simulink model "SecRwRtStHdrstUpwdDnwdTrgtPosSelc"  (R2018b)
settings: Solver=FixedStepDiscrete  StartTime=0.0  StopTime=10.0  FixedStep=0.01  RelTol=1e-3
undefined symbols (not defined in the file or in its folder): KeSMSw4SAcsMd23SecRwRtStHdrstUpwdDnwdPos_Val, KeSMSw4SAcsMd23SecRwRtStHdrstUpwdDnwdPosMax_Val, KeSMSw4SAcsMd23SecRwRtStHdrstUpwdDnwdPosMin_Val, KeSMSw4SAcsMd24SecRwRtStHdrstUpwdDnwdPos_Val, KeSMSw4SAcsMd24SecRwRtStHdrstUpwdDnwdPosMax_Val, KeSMSw4SAcsMd24SecRwRtStHdrstUpwdDnwdPosMin_Val, KeSMSw4SAcsMd25SecRwRtStHdrstUpwdDnwdPos_Val, KeSMSw4SAcsMd25SecRwRtStHdrstUpwdDnwdPosMax_Val, KeSMSw4SAcsMd25SecRwRtStHdrstUpwdDnwdPosMin_Val, KeSMSw4SAcsMd26SecRwRtStHdrstUpwdDnwdPos_Val, KeSMSw4SAcsMd26SecRwRtStHdrstUpwdDnwdPosMax_Val, KeSMSw4SAcsMd26SecRwRtStHdrstUpwdDnwdPosMin_Val, KeSMSw4sLyingMDSecRwRtStHdrstUpwdPos_160_Val, KeSMSw4sLyingMDSecRwRtStHdrstUpwdPos_165_Val, KeSMSw4sLyingMDSecRwRtStHdrstUpwdPos_170_Val, KeSMSw4sLyingMDSecRwRtStHdrstUpwdPos_175_Val, KeSMSw4sLyingMDSecRwRtStHdrstUpwdPos_180_Val, KeSMSw4sLyingMDSecRwRtStHdrstUpwdPos_Below160_Val, KeSMSw4sLyingMDSecRwRtStHdrstUpwdPos_Over180_Val, KeSMSw4sLyingMDSecRwRtStHdrstUpwdPosMax_160_Val, KeSMSw4sLyingMDSecRwRtStHdrstUpwdPosMax_165_Val, KeSMSw4sLyingMDSecRwRtStHdrstUpwdPosMax_170_Val, KeSMSw4sLyingMDSecRwRtStHdrstUpwdPosMax_175_Val, KeSMSw4sLyingMDSecRwRtStHdrstUpwdPosMax_180_Val, KeSMSw4sLyingMDSecRwRtStHdrstUpwdPosMax_Below160_Val, KeSMSw4sLyingMDSecRwRtStHdrstUpwdPosMax_Over180_Val, KeSMSw4sLyingMDSecRwRtStHdrstUpwdPosMin_160_Val, KeSMSw4sLyingMDSecRwRtStHdrstUpwdPosMin_165_Val, KeSMSw4sLyingMDSecRwRtStHdrstUpwdPosMin_170_Val, KeSMSw4sLyingMDSecRwRtStHdrstUpwdPosMin_175_Val, KeSMSw4sLyingMDSecRwRtStHdrstUpwdPosMin_180_Val, KeSMSw4sLyingMDSecRwRtStHdrstUpwdPosMin_Below160_Val, KeSMSw4sLyingMDSecRwRtStHdrstUpwdPosMin_Over180_Val, KeSMSw4sRecoveryMDSecRwRtStHdrstUpwdPos_160_Val, KeSMSw4sRecoveryMDSecRwRtStHdrstUpwdPos_165_Val, KeSMSw4sRecoveryMDSecRwRtStHdrstUpwdPos_170_Val, KeSMSw4sRecoveryMDSecRwRtStHdrstUpwdPos_175_Val, KeSMSw4sRecoveryMDSecRwRtStHdrstUpwdPos_180_Val, KeSMSw4sRecoveryMDSecRwRtStHdrstUpwdPos_Below160_Val, KeSMSw4sRecoveryMDSecRwRtStHdrstUpwdPos_Over180_Val, KeSMSw4sRecoveryMDSecRwRtStHdrstUpwdPosMax_160_Val, KeSMSw4sRecoveryMDSecRwRtStHdrstUpwdPosMax_165_Val, KeSMSw4sRecoveryMDSecRwRtStHdrstUpwdPosMax_170_Val, KeSMSw4sRecoveryMDSecRwRtStHdrstUpwdPosMax_175_Val, KeSMSw4sRecoveryMDSecRwRtStHdrstUpwdPosMax_180_Val, KeSMSw4sRecoveryMDSecRwRtStHdrstUpwdPosMax_Below160_Val, KeSMSw4sRecoveryMDSecRwRtStHdrstUpwdPosMax_Over180_Val, KeSMSw4sRecoveryMDSecRwRtStHdrstUpwdPosMin_160_Val, KeSMSw4sRecoveryMDSecRwRtStHdrstUpwdPosMin_165_Val, KeSMSw4sRecoveryMDSecRwRtStHdrstUpwdPosMin_170_Val, KeSMSw4sRecoveryMDSecRwRtStHdrstUpwdPosMin_175_Val, KeSMSw4sRecoveryMDSecRwRtStHdrstUpwdPosMin_180_Val, KeSMSw4sRecoveryMDSecRwRtStHdrstUpwdPosMin_Below160_Val, KeSMSw4sRecoveryMDSecRwRtStHdrstUpwdPosMin_Over180_Val, KeSMSw4sVIPMDSecRwRtStHdrstUpwdPos_160_Val, KeSMSw4sVIPMDSecRwRtStHdrstUpwdPos_165_Val, KeSMSw4sVIPMDSecRwRtStHdrstUpwdPos_170_Val, KeSMSw4sVIPMDSecRwRtStHdrstUpwdPos_175_Val, KeSMSw4sVIPMDSecRwRtStHdrstUpwdPos_180_Val, KeSMSw4sVIPMDSecRwRtStHdrstUpwdPos_Below160_Val ... (+15)
libraries: TrgtPosSelcLib x4
settings Model: ModifiedHistory=2023.8.1 V2.0.0 CR421790 增加模式21-26  Creator=sn2xws  LastModifiedBy=sn2xws
settings DataIOCC: SaveFormat=StructureWithTime
settings OptimizationCC: DefaultParameterBehavior=Inlined  EnhancedBackFolding=on  PassReuseOutputArgsAs=Individual arguments  ZeroExternalMemoryAtStartup=off  ZeroInternalMemoryAtStartup=off  OptimizeBlockOrder=speed  DifferentSizesBufferReuse=on  OptimizationCustomize=off
settings DebuggingCC: ParameterTunabilityLossMsg=error
settings ModelReferenceCC: ModelReferenceNumInstancesAllowed=Single
settings SFSimCC: MATLABDynamicMemAlloc=off
settings RTWCC: SystemTargetFile=autosar.tlc  GenCodeOnly=on  TemplateMakefile=ert_default_tmf  Description=AUTOSAR  GenerateReport=on  IncludeHyperlinkInReport=on  LaunchReport=on  GenerateTraceInfo=on  GenerateTraceReport=on  GenerateTraceReportSl=on  GenerateTraceReportSf=on  GenerateTraceReportEml=on
settings CodeAppCC: ForceParamTrailComments=on  IgnoreCustomStorageClasses=off  OperatorAnnotations=on  SimulinkDataObjDesc=on  SFDataObjDesc=on  InsertBlockDesc=on
settings STFCustomTargetCC: TargetLangStandard=C99 (ISO)  MultiwordLength=256  ParMdlRefBuildCompliant=on  CompOptLevelCompliant=on  IncludeMdlTerminateFcn=off  CombineOutputUpdateFcns=on  SuppressErrorStatus=on  ERTCustomFileBanners=on  SupportNonFinite=off  SupportComplex=off  SupportContinuousTime=off  SupportNonInlinedSFcns=off  RemoveResetFunc=on  MATLABClassNameForMDSCustomization=Simulink.SoftwareTarget.ERTCustomization  AutosarCompliant=on  UseToolchainInfoCompliant=on  LookupTableObjectStructAxisOrder=2,1,3,4,...  LUTObjectStructOrderEvenSpacing=Size,Table,Breakpoints  SystemTargetFile=autosar.tlc
settings ERTTargetCC: TargetLangStandard=C99 (ISO)  ConcurrentExecutionCompliant=off  IncludeMdlTerminateFcn=off  SuppressErrorStatus=on  SupportNonFinite=off  SupportComplex=off  ModelStepFunctionPrototypeControlCompliant=off  CPPClassGenCompliant=off  AutosarCompliant=on  LookupTableObjectStructAxisOrder=2,1,3,4,...  LUTObjectStructOrderEvenSpacing=Size,Table,Breakpoints  InlinedParameterPlacement=NonHierarchical  ERTCustomFileTemplate=example_file_process.tlc  ERTFilePackagingFormat=Compact

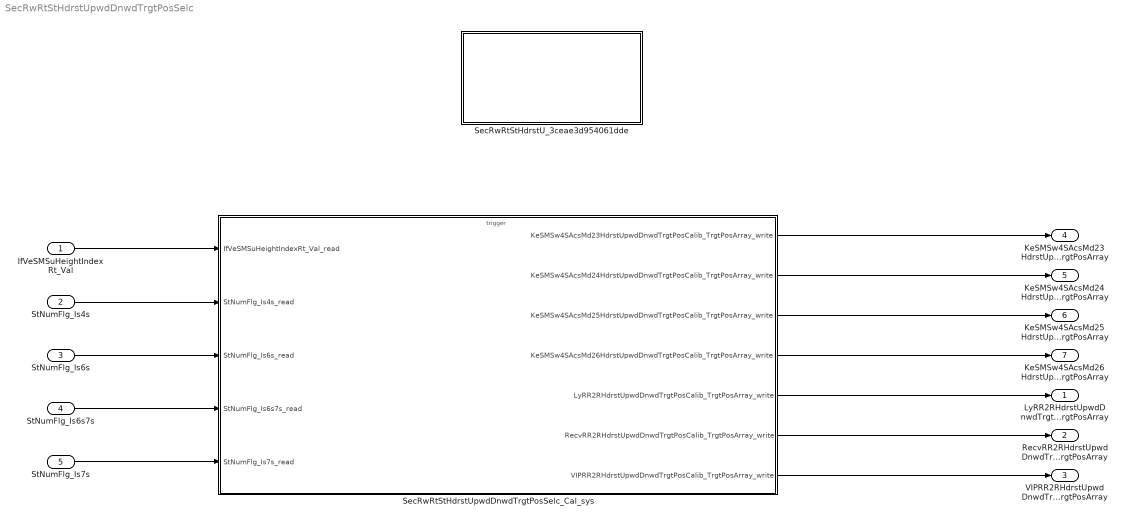
== system SecRwRtStHdrstUpwdDnwdTrgtPosSelc ==
  IfVeSMSuHeightIndexRt_Val : Inport  Description=|  OutDataTypeStr=uint8  PortDimensions=1
      | 0：under 160
      | 1：160
      | 2：165
      | 3：170
      | 4：175
      | 5：180
      | 6：over 180
  StNumFlg_Is4s : Inport  Port=2  OutDataTypeStr=boolean  PortDimensions=1
  StNumFlg_Is6s : Inport  Port=3  OutDataTypeStr=boolean  PortDimensions=1
  StNumFlg_Is6s7s : Inport  Port=4  OutDataTypeStr=boolean  PortDimensions=1
  StNumFlg_Is7s : Inport  Port=5  OutDataTypeStr=boolean  PortDimensions=1
  SecRwRtStHdrstU_3ceae3d954061dde : Subsystem
  SecRwRtStHdrstUpwdDnwdTrgtPosSelc_Cal_sys : Subsystem
  LyRR2RHdrstUpwdDnwdTrgtPosCalib_TrgtPosArray : Outport  Description=|  OutDataTypeStr=uint16  PortDimensions=3
      | 0:Pos
      | 1:Max
      | 2:Min
  RecvRR2RHdrstUpwdDnwdTrgtPosCalib_TrgtPosArray : Outport  Description=|  Port=2  OutDataTypeStr=uint16  PortDimensions=3
      | 0:Pos
      | 1:Max
      | 2:Min
  VIPRR2RHdrstUpwdDnwdTrgtPosCalib_TrgtPosArray : Outport  Description=|  Port=3  OutDataTypeStr=uint16  PortDimensions=3
      | 0:Pos
      | 1:Max
      | 2:Min
  KeSMSw4SAcsMd23HdrstUpwdDnwdTrgtPosCalib_TrgtPosArray : Outport  Description=|  Port=4  OutDataTypeStr=uint16  PortDimensions=3
      | 0:Pos
      | 1:Max
      | 2:Min
  KeSMSw4SAcsMd24HdrstUpwdDnwdTrgtPosCalib_TrgtPosArray : Outport  Description=|  Port=5  OutDataTypeStr=uint16  PortDimensions=3
      | 0:Pos
      | 1:Max
      | 2:Min
  KeSMSw4SAcsMd25HdrstUpwdDnwdTrgtPosCalib_TrgtPosArray : Outport  Description=|  Port=6  OutDataTypeStr=uint16  PortDimensions=3
      | 0:Pos
      | 1:Max
      | 2:Min
  KeSMSw4SAcsMd26HdrstUpwdDnwdTrgtPosCalib_TrgtPosArray : Outport  Description=|  Port=7  OutDataTypeStr=uint16  PortDimensions=3
      | 0:Pos
      | 1:Max
      | 2:Min
  wires:
  IfVeSMSuHeightIndexRt_Val/1 -> SecRwRtStHdrstUpwdDnwdTrgtPosSelc_Cal_sys/1(IfVeSMSuHeightIndexRt_Val_read)
  StNumFlg_Is4s/1 -> SecRwRtStHdrstUpwdDnwdTrgtPosSelc_Cal_sys/2(StNumFlg_Is4s_read)
  StNumFlg_Is6s/1 -> SecRwRtStHdrstUpwdDnwdTrgtPosSelc_Cal_sys/3(StNumFlg_Is6s_read)
  StNumFlg_Is6s7s/1 -> SecRwRtStHdrstUpwdDnwdTrgtPosSelc_Cal_sys/4(StNumFlg_Is6s7s_read)
  StNumFlg_Is7s/1 -> SecRwRtStHdrstUpwdDnwdTrgtPosSelc_Cal_sys/5(StNumFlg_Is7s_read)
  SecRwRtStHdrstUpwdDnwdTrgtPosSelc_Cal_sys/5(LyRR2RHdrstUpwdDnwdTrgtPosCalib_TrgtPosArray_write) -> LyRR2RHdrstUpwdDnwdTrgtPosCalib_TrgtPosArray/1
  SecRwRtStHdrstUpwdDnwdTrgtPosSelc_Cal_sys/6(RecvRR2RHdrstUpwdDnwdTrgtPosCalib_TrgtPosArray_write) -> RecvRR2RHdrstUpwdDnwdTrgtPosCalib_TrgtPosArray/1
  SecRwRtStHdrstUpwdDnwdTrgtPosSelc_Cal_sys/7(VIPRR2RHdrstUpwdDnwdTrgtPosCalib_TrgtPosArray_write) -> VIPRR2RHdrstUpwdDnwdTrgtPosCalib_TrgtPosArray/1
  SecRwRtStHdrstUpwdDnwdTrgtPosSelc_Cal_sys/1(KeSMSw4SAcsMd23HdrstUpwdDnwdTrgtPosCalib_TrgtPosArray_write) -> KeSMSw4SAcsMd23HdrstUpwdDnwdTrgtPosCalib_TrgtPosArray/1
  SecRwRtStHdrstUpwdDnwdTrgtPosSelc_Cal_sys/2(KeSMSw4SAcsMd24HdrstUpwdDnwdTrgtPosCalib_TrgtPosArray_write) -> KeSMSw4SAcsMd24HdrstUpwdDnwdTrgtPosCalib_TrgtPosArray/1
  SecRwRtStHdrstUpwdDnwdTrgtPosSelc_Cal_sys/3(KeSMSw4SAcsMd25HdrstUpwdDnwdTrgtPosCalib_TrgtPosArray_write) -> KeSMSw4SAcsMd25HdrstUpwdDnwdTrgtPosCalib_TrgtPosArray/1
  SecRwRtStHdrstUpwdDnwdTrgtPosSelc_Cal_sys/4(KeSMSw4SAcsMd26HdrstUpwdDnwdTrgtPosCalib_TrgtPosArray_write) -> KeSMSw4SAcsMd26HdrstUpwdDnwdTrgtPosCalib_TrgtPosArray/1

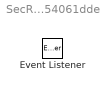
== system SecRwRtStHdrstUpwdDnwdTrgtPosSelc/SecRwRtStHdrstU_3ceae3d954061dde ==
  Event Listener : EventListener  EventName=reset

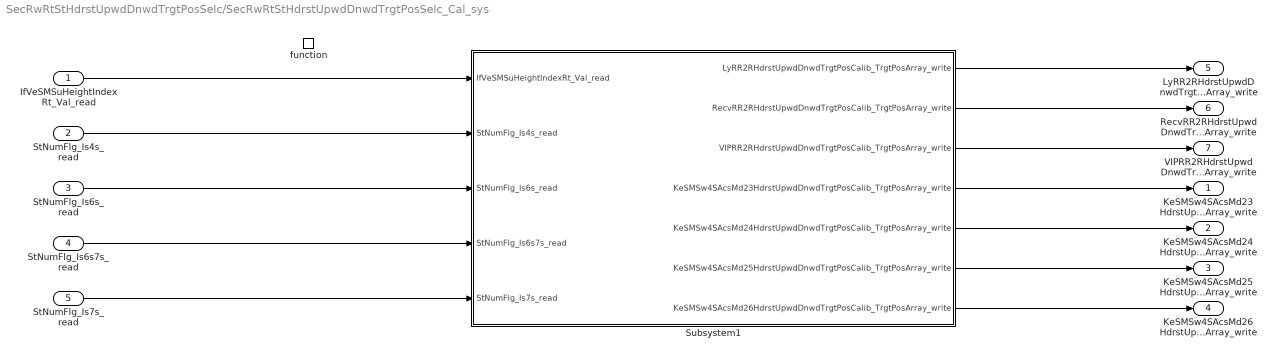
== system SecRwRtStHdrstUpwdDnwdTrgtPosSelc/SecRwRtStHdrstUpwdDnwdTrgtPosSelc_Cal_sys ==
  IfVeSMSuHeightIndexRt_Val_read : Inport
  StNumFlg_Is4s_read : Inport  Port=2
  StNumFlg_Is6s_read : Inport  Port=3
  StNumFlg_Is6s7s_read : Inport  Port=4
  StNumFlg_Is7s_read : Inport  Port=5
  function : TriggerPort  TriggerType=function-call  IsSimulinkFunction=on  FunctionName=SecRwRtStHdrstUpwdDnwdTrgtPosSelc_Cal  VariantControl=(inherit)
  Subsystem1 : Subsystem
  KeSMSw4SAcsMd23HdrstUpwdDnwdTrgtPosCalib_TrgtPosArray_write : Outport
      settings: EnsureOutportIsVirtual=on
  KeSMSw4SAcsMd24HdrstUpwdDnwdTrgtPosCalib_TrgtPosArray_write : Outport  Port=2
      settings: EnsureOutportIsVirtual=on
  KeSMSw4SAcsMd25HdrstUpwdDnwdTrgtPosCalib_TrgtPosArray_write : Outport  Port=3
      settings: EnsureOutportIsVirtual=on
  KeSMSw4SAcsMd26HdrstUpwdDnwdTrgtPosCalib_TrgtPosArray_write : Outport  Port=4
      settings: EnsureOutportIsVirtual=on
  LyRR2RHdrstUpwdDnwdTrgtPosCalib_TrgtPosArray_write : Outport  Port=5
      settings: EnsureOutportIsVirtual=on
  RecvRR2RHdrstUpwdDnwdTrgtPosCalib_TrgtPosArray_write : Outport  Port=6
      settings: EnsureOutportIsVirtual=on
  VIPRR2RHdrstUpwdDnwdTrgtPosCalib_TrgtPosArray_write : Outport  Port=7
      settings: EnsureOutportIsVirtual=on
  wires:
  Subsystem1/1(LyRR2RHdrstUpwdDnwdTrgtPosCalib_TrgtPosArray_write) -> LyRR2RHdrstUpwdDnwdTrgtPosCalib_TrgtPosArray_write/1
  Subsystem1/2(RecvRR2RHdrstUpwdDnwdTrgtPosCalib_TrgtPosArray_write) -> RecvRR2RHdrstUpwdDnwdTrgtPosCalib_TrgtPosArray_write/1
  Subsystem1/3(VIPRR2RHdrstUpwdDnwdTrgtPosCalib_TrgtPosArray_write) -> VIPRR2RHdrstUpwdDnwdTrgtPosCalib_TrgtPosArray_write/1
  Subsystem1/4(KeSMSw4SAcsMd23HdrstUpwdDnwdTrgtPosCalib_TrgtPosArray_write) -> KeSMSw4SAcsMd23HdrstUpwdDnwdTrgtPosCalib_TrgtPosArray_write/1
  Subsystem1/5(KeSMSw4SAcsMd24HdrstUpwdDnwdTrgtPosCalib_TrgtPosArray_write) -> KeSMSw4SAcsMd24HdrstUpwdDnwdTrgtPosCalib_TrgtPosArray_write/1
  Subsystem1/6(KeSMSw4SAcsMd25HdrstUpwdDnwdTrgtPosCalib_TrgtPosArray_write) -> KeSMSw4SAcsMd25HdrstUpwdDnwdTrgtPosCalib_TrgtPosArray_write/1
  Subsystem1/7(KeSMSw4SAcsMd26HdrstUpwdDnwdTrgtPosCalib_TrgtPosArray_write) -> KeSMSw4SAcsMd26HdrstUpwdDnwdTrgtPosCalib_TrgtPosArray_write/1
  StNumFlg_Is6s7s_read/1 -> Subsystem1/4(StNumFlg_Is6s7s_read)
  StNumFlg_Is6s_read/1 -> Subsystem1/3(StNumFlg_Is6s_read)
  StNumFlg_Is7s_read/1 -> Subsystem1/5(StNumFlg_Is7s_read)
  StNumFlg_Is4s_read/1 -> Subsystem1/2(StNumFlg_Is4s_read)
  IfVeSMSuHeightIndexRt_Val_read/1 -> Subsystem1/1(IfVeSMSuHeightIndexRt_Val_read)

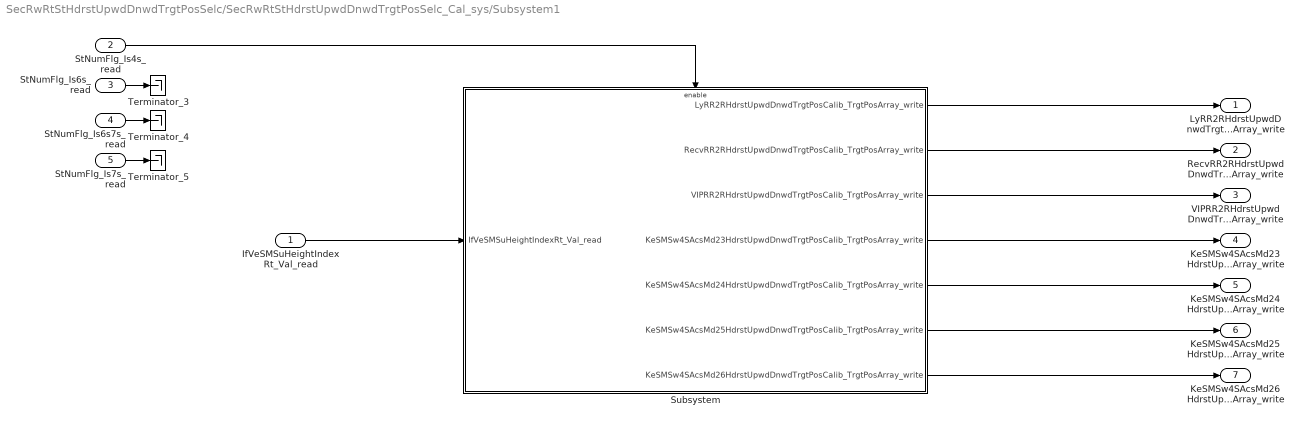
== system SecRwRtStHdrstUpwdDnwdTrgtPosSelc/SecRwRtStHdrstUpwdDnwdTrgtPosSelc_Cal_sys/Subsystem1 ==
  IfVeSMSuHeightIndexRt_Val_read : Inport
  StNumFlg_Is4s_read : Inport  Port=2
  StNumFlg_Is6s_read : Inport  Port=3
  StNumFlg_Is6s7s_read : Inport  Port=4
  StNumFlg_Is7s_read : Inport  Port=5
  Subsystem : Subsystem
  Terminator_3 : Terminator
  Terminator_4 : Terminator
  Terminator_5 : Terminator
  LyRR2RHdrstUpwdDnwdTrgtPosCalib_TrgtPosArray_write : Outport
      settings: EnsureOutportIsVirtual=on
  RecvRR2RHdrstUpwdDnwdTrgtPosCalib_TrgtPosArray_write : Outport  Port=2
      settings: EnsureOutportIsVirtual=on
  VIPRR2RHdrstUpwdDnwdTrgtPosCalib_TrgtPosArray_write : Outport  Port=3
      settings: EnsureOutportIsVirtual=on
  KeSMSw4SAcsMd23HdrstUpwdDnwdTrgtPosCalib_TrgtPosArray_write : Outport  Port=4
      settings: EnsureOutportIsVirtual=on
  KeSMSw4SAcsMd24HdrstUpwdDnwdTrgtPosCalib_TrgtPosArray_write : Outport  Port=5
      settings: EnsureOutportIsVirtual=on
  KeSMSw4SAcsMd25HdrstUpwdDnwdTrgtPosCalib_TrgtPosArray_write : Outport  Port=6
      settings: EnsureOutportIsVirtual=on
  KeSMSw4SAcsMd26HdrstUpwdDnwdTrgtPosCalib_TrgtPosArray_write : Outport  Port=7
      settings: EnsureOutportIsVirtual=on
  wires:
  Subsystem/3(VIPRR2RHdrstUpwdDnwdTrgtPosCalib_TrgtPosArray_write) -> VIPRR2RHdrstUpwdDnwdTrgtPosCalib_TrgtPosArray_write/1
  IfVeSMSuHeightIndexRt_Val_read/1 -> Subsystem/1(IfVeSMSuHeightIndexRt_Val_read)
  StNumFlg_Is4s_read/1 -> Subsystem/Enable
  StNumFlg_Is7s_read/1 -> Terminator_5/1
  StNumFlg_Is6s_read/1 -> Terminator_3/1
  StNumFlg_Is6s7s_read/1 -> Terminator_4/1
  Subsystem/2(RecvRR2RHdrstUpwdDnwdTrgtPosCalib_TrgtPosArray_write) -> RecvRR2RHdrstUpwdDnwdTrgtPosCalib_TrgtPosArray_write/1
  Subsystem/1(LyRR2RHdrstUpwdDnwdTrgtPosCalib_TrgtPosArray_write) -> LyRR2RHdrstUpwdDnwdTrgtPosCalib_TrgtPosArray_write/1
  Subsystem/4(KeSMSw4SAcsMd23HdrstUpwdDnwdTrgtPosCalib_TrgtPosArray_write) -> KeSMSw4SAcsMd23HdrstUpwdDnwdTrgtPosCalib_TrgtPosArray_write/1
  Subsystem/5(KeSMSw4SAcsMd24HdrstUpwdDnwdTrgtPosCalib_TrgtPosArray_write) -> KeSMSw4SAcsMd24HdrstUpwdDnwdTrgtPosCalib_TrgtPosArray_write/1
  Subsystem/6(KeSMSw4SAcsMd25HdrstUpwdDnwdTrgtPosCalib_TrgtPosArray_write) -> KeSMSw4SAcsMd25HdrstUpwdDnwdTrgtPosCalib_TrgtPosArray_write/1
  Subsystem/7(KeSMSw4SAcsMd26HdrstUpwdDnwdTrgtPosCalib_TrgtPosArray_write) -> KeSMSw4SAcsMd26HdrstUpwdDnwdTrgtPosCalib_TrgtPosArray_write/1

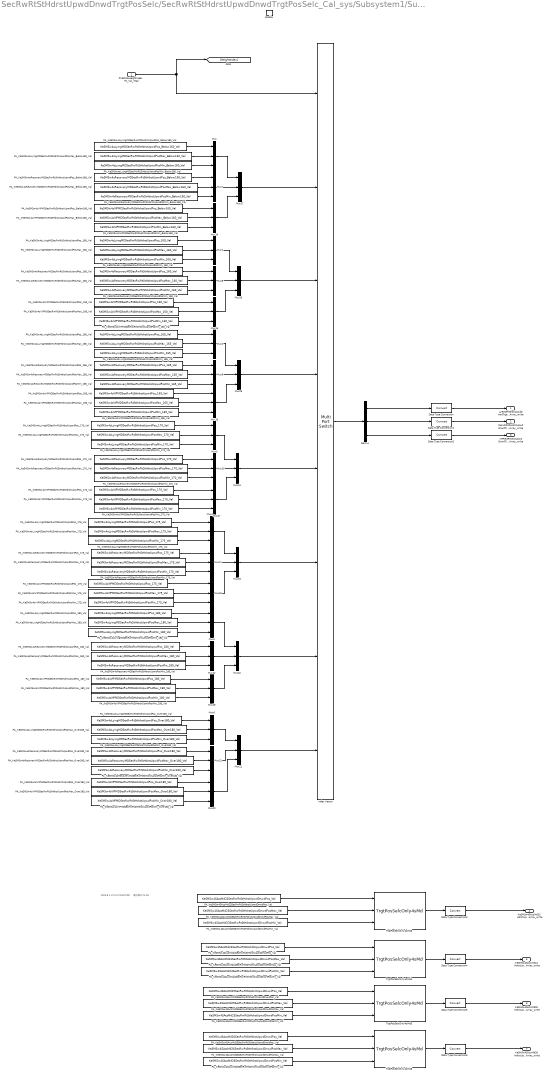
== system SecRwRtStHdrstUpwdDnwdTrgtPosSelc/SecRwRtStHdrstUpwdDnwdTrgtPosSelc_Cal_sys/Subsystem1/Subsystem ==
  note: 2023.8.1 V2.0.0 CR401790 增加模式21-26
  IfVeSMSuHeightIndexRt_Val_read : Inport
  Enable : EnablePort
  Data Type Conversion{,1..6} (7 alike) : DataTypeConversion
  Demux : Demux  Outputs=3
  Index Vector : MultiPortSwitch  DataPortOrder=Zero-based contiguous  Inputs=7  zeroidx=on
  Mux{,1..27} (28 alike) : Mux  Inputs=3
  PA_KeSMSw4SAcsMd23SecRwRtStHdrstUpwdDnwdPosMax_Val : Constant  Value=KeSMSw4SAcsMd23SecRwRtStHdrstUpwdDnwdPosMax_Val
  PA_KeSMSw4SAcsMd23SecRwRtStHdrstUpwdDnwdPosMin_Val : Constant  Value=KeSMSw4SAcsMd23SecRwRtStHdrstUpwdDnwdPosMin_Val
  PA_KeSMSw4SAcsMd23SecRwRtStHdrstUpwdDnwdPos_Val : Constant  Value=KeSMSw4SAcsMd23SecRwRtStHdrstUpwdDnwdPos_Val
  PA_KeSMSw4SAcsMd24SecRwRtStHdrstUpwdDnwdPosMax_Val : Constant  Value=KeSMSw4SAcsMd24SecRwRtStHdrstUpwdDnwdPosMax_Val
  PA_KeSMSw4SAcsMd24SecRwRtStHdrstUpwdDnwdPosMin_Val : Constant  Value=KeSMSw4SAcsMd24SecRwRtStHdrstUpwdDnwdPosMin_Val
  PA_KeSMSw4SAcsMd24SecRwRtStHdrstUpwdDnwdPos_Val : Constant  Value=KeSMSw4SAcsMd24SecRwRtStHdrstUpwdDnwdPos_Val
  PA_KeSMSw4SAcsMd25SecRwRtStHdrstUpwdDnwdPosMax_Val : Constant  Value=KeSMSw4SAcsMd25SecRwRtStHdrstUpwdDnwdPosMax_Val
  PA_KeSMSw4SAcsMd25SecRwRtStHdrstUpwdDnwdPosMin_Val : Constant  Value=KeSMSw4SAcsMd25SecRwRtStHdrstUpwdDnwdPosMin_Val
  PA_KeSMSw4SAcsMd25SecRwRtStHdrstUpwdDnwdPos_Val : Constant  Value=KeSMSw4SAcsMd25SecRwRtStHdrstUpwdDnwdPos_Val
  PA_KeSMSw4SAcsMd26SecRwRtStHdrstUpwdDnwdPosMax_Val : Constant  Value=KeSMSw4SAcsMd26SecRwRtStHdrstUpwdDnwdPosMax_Val
  PA_KeSMSw4SAcsMd26SecRwRtStHdrstUpwdDnwdPosMin_Val : Constant  Value=KeSMSw4SAcsMd26SecRwRtStHdrstUpwdDnwdPosMin_Val
  PA_KeSMSw4SAcsMd26SecRwRtStHdrstUpwdDnwdPos_Val : Constant  Value=KeSMSw4SAcsMd26SecRwRtStHdrstUpwdDnwdPos_Val
  PA_KeSMSw4sLyingMDSecRwRtStHdrstUpwdPosMax_160_Val : Constant  Value=KeSMSw4sLyingMDSecRwRtStHdrstUpwdPosMax_160_Val
  PA_KeSMSw4sLyingMDSecRwRtStHdrstUpwdPosMax_165_Val : Constant  Value=KeSMSw4sLyingMDSecRwRtStHdrstUpwdPosMax_165_Val
  PA_KeSMSw4sLyingMDSecRwRtStHdrstUpwdPosMax_170_Val : Constant  Value=KeSMSw4sLyingMDSecRwRtStHdrstUpwdPosMax_170_Val
  PA_KeSMSw4sLyingMDSecRwRtStHdrstUpwdPosMax_175_Val : Constant  Value=KeSMSw4sLyingMDSecRwRtStHdrstUpwdPosMax_175_Val
  PA_KeSMSw4sLyingMDSecRwRtStHdrstUpwdPosMax_180_Val : Constant  Value=KeSMSw4sLyingMDSecRwRtStHdrstUpwdPosMax_180_Val
  PA_KeSMSw4sLyingMDSecRwRtStHdrstUpwdPosMax_Below160_Val : Constant  Value=KeSMSw4sLyingMDSecRwRtStHdrstUpwdPosMax_Below160_Val
  PA_KeSMSw4sLyingMDSecRwRtStHdrstUpwdPosMax_Over180_Val : Constant  Value=KeSMSw4sLyingMDSecRwRtStHdrstUpwdPosMax_Over180_Val
  PA_KeSMSw4sLyingMDSecRwRtStHdrstUpwdPosMin_160_Val : Constant  Value=KeSMSw4sLyingMDSecRwRtStHdrstUpwdPosMin_160_Val
  PA_KeSMSw4sLyingMDSecRwRtStHdrstUpwdPosMin_165_Val : Constant  Value=KeSMSw4sLyingMDSecRwRtStHdrstUpwdPosMin_165_Val
  PA_KeSMSw4sLyingMDSecRwRtStHdrstUpwdPosMin_170_Val : Constant  Value=KeSMSw4sLyingMDSecRwRtStHdrstUpwdPosMin_170_Val
  PA_KeSMSw4sLyingMDSecRwRtStHdrstUpwdPosMin_175_Val : Constant  Value=KeSMSw4sLyingMDSecRwRtStHdrstUpwdPosMin_175_Val
  PA_KeSMSw4sLyingMDSecRwRtStHdrstUpwdPosMin_180_Val : Constant  Value=KeSMSw4sLyingMDSecRwRtStHdrstUpwdPosMin_180_Val
  PA_KeSMSw4sLyingMDSecRwRtStHdrstUpwdPosMin_Below160_Val : Constant  Value=KeSMSw4sLyingMDSecRwRtStHdrstUpwdPosMin_Below160_Val
  PA_KeSMSw4sLyingMDSecRwRtStHdrstUpwdPosMin_Over180_Val : Constant  Value=KeSMSw4sLyingMDSecRwRtStHdrstUpwdPosMin_Over180_Val
  PA_KeSMSw4sLyingMDSecRwRtStHdrstUpwdPos_160_Val : Constant  Value=KeSMSw4sLyingMDSecRwRtStHdrstUpwdPos_160_Val
  PA_KeSMSw4sLyingMDSecRwRtStHdrstUpwdPos_165_Val : Constant  Value=KeSMSw4sLyingMDSecRwRtStHdrstUpwdPos_165_Val
  PA_KeSMSw4sLyingMDSecRwRtStHdrstUpwdPos_170_Val : Constant  Value=KeSMSw4sLyingMDSecRwRtStHdrstUpwdPos_170_Val
  PA_KeSMSw4sLyingMDSecRwRtStHdrstUpwdPos_175_Val : Constant  Value=KeSMSw4sLyingMDSecRwRtStHdrstUpwdPos_175_Val
  PA_KeSMSw4sLyingMDSecRwRtStHdrstUpwdPos_180_Val : Constant  Value=KeSMSw4sLyingMDSecRwRtStHdrstUpwdPos_180_Val
  PA_KeSMSw4sLyingMDSecRwRtStHdrstUpwdPos_Below160_Val : Constant  Value=KeSMSw4sLyingMDSecRwRtStHdrstUpwdPos_Below160_Val
  PA_KeSMSw4sLyingMDSecRwRtStHdrstUpwdPos_Over180_Val : Constant  Value=KeSMSw4sLyingMDSecRwRtStHdrstUpwdPos_Over180_Val
  PA_KeSMSw4sRecoveryMDSecRwRtStHdrstUpwdPosMax_160_Val : Constant  Value=KeSMSw4sRecoveryMDSecRwRtStHdrstUpwdPosMax_160_Val
  PA_KeSMSw4sRecoveryMDSecRwRtStHdrstUpwdPosMax_165_Val : Constant  Value=KeSMSw4sRecoveryMDSecRwRtStHdrstUpwdPosMax_165_Val
  PA_KeSMSw4sRecoveryMDSecRwRtStHdrstUpwdPosMax_170_Val : Constant  Value=KeSMSw4sRecoveryMDSecRwRtStHdrstUpwdPosMax_170_Val
  PA_KeSMSw4sRecoveryMDSecRwRtStHdrstUpwdPosMax_175_Val : Constant  Value=KeSMSw4sRecoveryMDSecRwRtStHdrstUpwdPosMax_175_Val
  PA_KeSMSw4sRecoveryMDSecRwRtStHdrstUpwdPosMax_180_Val : Constant  Value=KeSMSw4sRecoveryMDSecRwRtStHdrstUpwdPosMax_180_Val
  PA_KeSMSw4sRecoveryMDSecRwRtStHdrstUpwdPosMax_Below160_Val : Constant  Value=KeSMSw4sRecoveryMDSecRwRtStHdrstUpwdPosMax_Below160_Val
  PA_KeSMSw4sRecoveryMDSecRwRtStHdrstUpwdPosMax_Over180_Val : Constant  Value=KeSMSw4sRecoveryMDSecRwRtStHdrstUpwdPosMax_Over180_Val
  PA_KeSMSw4sRecoveryMDSecRwRtStHdrstUpwdPosMin_160_Val : Constant  Value=KeSMSw4sRecoveryMDSecRwRtStHdrstUpwdPosMin_160_Val
  PA_KeSMSw4sRecoveryMDSecRwRtStHdrstUpwdPosMin_165_Val : Constant  Value=KeSMSw4sRecoveryMDSecRwRtStHdrstUpwdPosMin_165_Val
  PA_KeSMSw4sRecoveryMDSecRwRtStHdrstUpwdPosMin_170_Val : Constant  Value=KeSMSw4sRecoveryMDSecRwRtStHdrstUpwdPosMin_170_Val
  PA_KeSMSw4sRecoveryMDSecRwRtStHdrstUpwdPosMin_175_Val : Constant  Value=KeSMSw4sRecoveryMDSecRwRtStHdrstUpwdPosMin_175_Val
  PA_KeSMSw4sRecoveryMDSecRwRtStHdrstUpwdPosMin_180_Val : Constant  Value=KeSMSw4sRecoveryMDSecRwRtStHdrstUpwdPosMin_180_Val
  PA_KeSMSw4sRecoveryMDSecRwRtStHdrstUpwdPosMin_Below160_Val : Constant  Value=KeSMSw4sRecoveryMDSecRwRtStHdrstUpwdPosMin_Below160_Val
  PA_KeSMSw4sRecoveryMDSecRwRtStHdrstUpwdPosMin_Over180_Val : Constant  Value=KeSMSw4sRecoveryMDSecRwRtStHdrstUpwdPosMin_Over180_Val
  PA_KeSMSw4sRecoveryMDSecRwRtStHdrstUpwdPos_160_Val : Constant  Value=KeSMSw4sRecoveryMDSecRwRtStHdrstUpwdPos_160_Val
  PA_KeSMSw4sRecoveryMDSecRwRtStHdrstUpwdPos_165_Val : Constant  Value=KeSMSw4sRecoveryMDSecRwRtStHdrstUpwdPos_165_Val
  PA_KeSMSw4sRecoveryMDSecRwRtStHdrstUpwdPos_170_Val : Constant  Value=KeSMSw4sRecoveryMDSecRwRtStHdrstUpwdPos_170_Val
  PA_KeSMSw4sRecoveryMDSecRwRtStHdrstUpwdPos_175_Val : Constant  Value=KeSMSw4sRecoveryMDSecRwRtStHdrstUpwdPos_175_Val
  PA_KeSMSw4sRecoveryMDSecRwRtStHdrstUpwdPos_180_Val : Constant  Value=KeSMSw4sRecoveryMDSecRwRtStHdrstUpwdPos_180_Val
  PA_KeSMSw4sRecoveryMDSecRwRtStHdrstUpwdPos_Below160_Val : Constant  Value=KeSMSw4sRecoveryMDSecRwRtStHdrstUpwdPos_Below160_Val
  PA_KeSMSw4sRecoveryMDSecRwRtStHdrstUpwdPos_Over180_Val : Constant  Value=KeSMSw4sRecoveryMDSecRwRtStHdrstUpwdPos_Over180_Val
  PA_KeSMSw4sVIPMDSecRwRtStHdrstUpwdPosMax_160_Val : Constant  Value=KeSMSw4sVIPMDSecRwRtStHdrstUpwdPosMax_160_Val
  PA_KeSMSw4sVIPMDSecRwRtStHdrstUpwdPosMax_165_Val : Constant  Value=KeSMSw4sVIPMDSecRwRtStHdrstUpwdPosMax_165_Val
  PA_KeSMSw4sVIPMDSecRwRtStHdrstUpwdPosMax_170_Val : Constant  Value=KeSMSw4sVIPMDSecRwRtStHdrstUpwdPosMax_170_Val
  PA_KeSMSw4sVIPMDSecRwRtStHdrstUpwdPosMax_175_Val : Constant  Value=KeSMSw4sVIPMDSecRwRtStHdrstUpwdPosMax_175_Val
  PA_KeSMSw4sVIPMDSecRwRtStHdrstUpwdPosMax_180_Val : Constant  Value=KeSMSw4sVIPMDSecRwRtStHdrstUpwdPosMax_180_Val
  PA_KeSMSw4sVIPMDSecRwRtStHdrstUpwdPosMax_Below160_Val : Constant  Value=KeSMSw4sVIPMDSecRwRtStHdrstUpwdPosMax_Below160_Val
  PA_KeSMSw4sVIPMDSecRwRtStHdrstUpwdPosMax_Over180_Val : Constant  Value=KeSMSw4sVIPMDSecRwRtStHdrstUpwdPosMax_Over180_Val
  PA_KeSMSw4sVIPMDSecRwRtStHdrstUpwdPosMin_160_Val : Constant  Value=KeSMSw4sVIPMDSecRwRtStHdrstUpwdPosMin_160_Val
  PA_KeSMSw4sVIPMDSecRwRtStHdrstUpwdPosMin_165_Val : Constant  Value=KeSMSw4sVIPMDSecRwRtStHdrstUpwdPosMin_165_Val
  PA_KeSMSw4sVIPMDSecRwRtStHdrstUpwdPosMin_170_Val : Constant  Value=KeSMSw4sVIPMDSecRwRtStHdrstUpwdPosMin_170_Val
  PA_KeSMSw4sVIPMDSecRwRtStHdrstUpwdPosMin_175_Val : Constant  Value=KeSMSw4sVIPMDSecRwRtStHdrstUpwdPosMin_175_Val
  PA_KeSMSw4sVIPMDSecRwRtStHdrstUpwdPosMin_180_Val : Constant  Value=KeSMSw4sVIPMDSecRwRtStHdrstUpwdPosMin_180_Val
  PA_KeSMSw4sVIPMDSecRwRtStHdrstUpwdPosMin_Below160_Val : Constant  Value=KeSMSw4sVIPMDSecRwRtStHdrstUpwdPosMin_Below160_Val
  PA_KeSMSw4sVIPMDSecRwRtStHdrstUpwdPosMin_Over180_Val : Constant  Value=KeSMSw4sVIPMDSecRwRtStHdrstUpwdPosMin_Over180_Val
  PA_KeSMSw4sVIPMDSecRwRtStHdrstUpwdPos_160_Val : Constant  Value=KeSMSw4sVIPMDSecRwRtStHdrstUpwdPos_160_Val
  PA_KeSMSw4sVIPMDSecRwRtStHdrstUpwdPos_165_Val : Constant  Value=KeSMSw4sVIPMDSecRwRtStHdrstUpwdPos_165_Val
  PA_KeSMSw4sVIPMDSecRwRtStHdrstUpwdPos_170_Val : Constant  Value=KeSMSw4sVIPMDSecRwRtStHdrstUpwdPos_170_Val
  PA_KeSMSw4sVIPMDSecRwRtStHdrstUpwdPos_175_Val : Constant  Value=KeSMSw4sVIPMDSecRwRtStHdrstUpwdPos_175_Val
  PA_KeSMSw4sVIPMDSecRwRtStHdrstUpwdPos_180_Val : Constant  Value=KeSMSw4sVIPMDSecRwRtStHdrstUpwdPos_180_Val
  PA_KeSMSw4sVIPMDSecRwRtStHdrstUpwdPos_Below160_Val : Constant  Value=KeSMSw4sVIPMDSecRwRtStHdrstUpwdPos_Below160_Val
  PA_KeSMSw4sVIPMDSecRwRtStHdrstUpwdPos_Over180_Val : Constant  Value=KeSMSw4sVIPMDSecRwRtStHdrstUpwdPos_Over180_Val
  TrgtPosSelcOnly4sMd{3..6} (4 alike) : TrgtPosSelcLib/TrgtPosSelcOnly4sMd  SystemSampleTime=-1
  LyRR2RHdrstUpwdDnwdTrgtPosCalib_TrgtPosArray_write : Outport
  RecvRR2RHdrstUpwdDnwdTrgtPosCalib_TrgtPosArray_write : Outport  Port=2
  VIPRR2RHdrstUpwdDnwdTrgtPosCalib_TrgtPosArray_write : Outport  Port=3
  KeSMSw4SAcsMd23HdrstUpwdDnwdTrgtPosCalib_TrgtPosArray_write : Outport  Port=4
  KeSMSw4SAcsMd24HdrstUpwdDnwdTrgtPosCalib_TrgtPosArray_write : Outport  Port=5
  KeSMSw4SAcsMd25HdrstUpwdDnwdTrgtPosCalib_TrgtPosArray_write : Outport  Port=6
  KeSMSw4SAcsMd26HdrstUpwdDnwdTrgtPosCalib_TrgtPosArray_write : Outport  Port=7
  wires:
  Demux/1 -> Data Type Conversion/1
  IfVeSMSuHeightIndexRt_Val_read/1 -> [HeightIndex], Index Vector/1
  Demux/2 -> Data Type Conversion1/1
  Demux/3 -> Data Type Conversion2/1
  Data Type Conversion/1 -> LyRR2RHdrstUpwdDnwdTrgtPosCalib_TrgtPosArray_write/1
  Data Type Conversion1/1 -> RecvRR2RHdrstUpwdDnwdTrgtPosCalib_TrgtPosArray_write/1
  Data Type Conversion2/1 -> VIPRR2RHdrstUpwdDnwdTrgtPosCalib_TrgtPosArray_write/1
  PA_KeSMSw4SAcsMd23SecRwRtStHdrstUpwdDnwdPos_Val/1 -> TrgtPosSelcOnly4sMd3/1
  PA_KeSMSw4SAcsMd24SecRwRtStHdrstUpwdDnwdPos_Val/1 -> TrgtPosSelcOnly4sMd4/1
  PA_KeSMSw4SAcsMd25SecRwRtStHdrstUpwdDnwdPos_Val/1 -> TrgtPosSelcOnly4sMd5/1
  PA_KeSMSw4SAcsMd26SecRwRtStHdrstUpwdDnwdPos_Val/1 -> TrgtPosSelcOnly4sMd6/1
  TrgtPosSelcOnly4sMd5/1 -> Data Type Conversion5/1
  TrgtPosSelcOnly4sMd6/1 -> Data Type Conversion6/1
  TrgtPosSelcOnly4sMd3/1 -> Data Type Conversion3/1
  TrgtPosSelcOnly4sMd4/1 -> Data Type Conversion4/1
  PA_KeSMSw4SAcsMd23SecRwRtStHdrstUpwdDnwdPosMax_Val/1 -> TrgtPosSelcOnly4sMd3/2
  PA_KeSMSw4SAcsMd23SecRwRtStHdrstUpwdDnwdPosMin_Val/1 -> TrgtPosSelcOnly4sMd3/3
  PA_KeSMSw4SAcsMd24SecRwRtStHdrstUpwdDnwdPosMax_Val/1 -> TrgtPosSelcOnly4sMd4/2
  PA_KeSMSw4SAcsMd24SecRwRtStHdrstUpwdDnwdPosMin_Val/1 -> TrgtPosSelcOnly4sMd4/3
  PA_KeSMSw4SAcsMd25SecRwRtStHdrstUpwdDnwdPosMax_Val/1 -> TrgtPosSelcOnly4sMd5/2
  PA_KeSMSw4SAcsMd25SecRwRtStHdrstUpwdDnwdPosMin_Val/1 -> TrgtPosSelcOnly4sMd5/3
  PA_KeSMSw4SAcsMd26SecRwRtStHdrstUpwdDnwdPosMax_Val/1 -> TrgtPosSelcOnly4sMd6/2
  PA_KeSMSw4SAcsMd26SecRwRtStHdrstUpwdDnwdPosMin_Val/1 -> TrgtPosSelcOnly4sMd6/3
  Data Type Conversion3/1 -> KeSMSw4SAcsMd23HdrstUpwdDnwdTrgtPosCalib_TrgtPosArray_write/1
  Data Type Conversion4/1 -> KeSMSw4SAcsMd24HdrstUpwdDnwdTrgtPosCalib_TrgtPosArray_write/1
  Data Type Conversion5/1 -> KeSMSw4SAcsMd25HdrstUpwdDnwdTrgtPosCalib_TrgtPosArray_write/1
  Data Type Conversion6/1 -> KeSMSw4SAcsMd26HdrstUpwdDnwdTrgtPosCalib_TrgtPosArray_write/1
  PA_KeSMSw4sLyingMDSecRwRtStHdrstUpwdPos_Below160_Val/1 -> Mux/1
  PA_KeSMSw4sLyingMDSecRwRtStHdrstUpwdPosMax_Below160_Val/1 -> Mux/2
  PA_KeSMSw4sLyingMDSecRwRtStHdrstUpwdPosMin_Below160_Val/1 -> Mux/3
  PA_KeSMSw4sLyingMDSecRwRtStHdrstUpwdPosMax_160_Val/1 -> Mux1/2
  PA_KeSMSw4sLyingMDSecRwRtStHdrstUpwdPosMin_160_Val/1 -> Mux1/3
  PA_KeSMSw4sLyingMDSecRwRtStHdrstUpwdPos_160_Val/1 -> Mux1/1
  PA_KeSMSw4sLyingMDSecRwRtStHdrstUpwdPosMax_165_Val/1 -> Mux2/2
  PA_KeSMSw4sLyingMDSecRwRtStHdrstUpwdPosMin_165_Val/1 -> Mux2/3
  PA_KeSMSw4sLyingMDSecRwRtStHdrstUpwdPos_165_Val/1 -> Mux2/1
  PA_KeSMSw4sLyingMDSecRwRtStHdrstUpwdPosMax_170_Val/1 -> Mux3/2
  PA_KeSMSw4sLyingMDSecRwRtStHdrstUpwdPosMin_170_Val/1 -> Mux3/3
  PA_KeSMSw4sLyingMDSecRwRtStHdrstUpwdPos_170_Val/1 -> Mux3/1
  PA_KeSMSw4sLyingMDSecRwRtStHdrstUpwdPosMax_175_Val/1 -> Mux4/2
  PA_KeSMSw4sLyingMDSecRwRtStHdrstUpwdPosMin_175_Val/1 -> Mux4/3
  PA_KeSMSw4sLyingMDSecRwRtStHdrstUpwdPos_175_Val/1 -> Mux4/1
  PA_KeSMSw4sLyingMDSecRwRtStHdrstUpwdPosMax_180_Val/1 -> Mux5/2
  PA_KeSMSw4sLyingMDSecRwRtStHdrstUpwdPos_180_Val/1 -> Mux5/1
  PA_KeSMSw4sLyingMDSecRwRtStHdrstUpwdPosMin_180_Val/1 -> Mux5/3
  PA_KeSMSw4sLyingMDSecRwRtStHdrstUpwdPosMax_Over180_Val/1 -> Mux6/2
  PA_KeSMSw4sLyingMDSecRwRtStHdrstUpwdPosMin_Over180_Val/1 -> Mux6/3
  PA_KeSMSw4sLyingMDSecRwRtStHdrstUpwdPos_Over180_Val/1 -> Mux6/1
  PA_KeSMSw4sRecoveryMDSecRwRtStHdrstUpwdPosMax_Below160_Val/1 -> Mux7/2
  PA_KeSMSw4sRecoveryMDSecRwRtStHdrstUpwdPosMin_Below160_Val/1 -> Mux7/3
  PA_KeSMSw4sRecoveryMDSecRwRtStHdrstUpwdPos_Below160_Val/1 -> Mux7/1
  PA_KeSMSw4sRecoveryMDSecRwRtStHdrstUpwdPosMax_160_Val/1 -> Mux8/2
  PA_KeSMSw4sRecoveryMDSecRwRtStHdrstUpwdPosMin_160_Val/1 -> Mux8/3
  PA_KeSMSw4sRecoveryMDSecRwRtStHdrstUpwdPos_160_Val/1 -> Mux8/1
  PA_KeSMSw4sRecoveryMDSecRwRtStHdrstUpwdPosMax_165_Val/1 -> Mux9/2
  PA_KeSMSw4sRecoveryMDSecRwRtStHdrstUpwdPosMin_165_Val/1 -> Mux9/3
  PA_KeSMSw4sRecoveryMDSecRwRtStHdrstUpwdPos_165_Val/1 -> Mux9/1
  PA_KeSMSw4sRecoveryMDSecRwRtStHdrstUpwdPosMax_170_Val/1 -> Mux10/2
  PA_KeSMSw4sRecoveryMDSecRwRtStHdrstUpwdPosMin_170_Val/1 -> Mux10/3
  PA_KeSMSw4sRecoveryMDSecRwRtStHdrstUpwdPos_170_Val/1 -> Mux10/1
  PA_KeSMSw4sRecoveryMDSecRwRtStHdrstUpwdPosMax_175_Val/1 -> Mux11/2
  PA_KeSMSw4sRecoveryMDSecRwRtStHdrstUpwdPosMin_175_Val/1 -> Mux11/3
  PA_KeSMSw4sRecoveryMDSecRwRtStHdrstUpwdPos_175_Val/1 -> Mux11/1
  PA_KeSMSw4sRecoveryMDSecRwRtStHdrstUpwdPosMax_180_Val/1 -> Mux12/2
  PA_KeSMSw4sRecoveryMDSecRwRtStHdrstUpwdPosMin_180_Val/1 -> Mux12/3
  PA_KeSMSw4sRecoveryMDSecRwRtStHdrstUpwdPos_180_Val/1 -> Mux12/1
  PA_KeSMSw4sRecoveryMDSecRwRtStHdrstUpwdPosMax_Over180_Val/1 -> Mux13/2
  PA_KeSMSw4sRecoveryMDSecRwRtStHdrstUpwdPosMin_Over180_Val/1 -> Mux13/3
  PA_KeSMSw4sRecoveryMDSecRwRtStHdrstUpwdPos_Over180_Val/1 -> Mux13/1
  PA_KeSMSw4sVIPMDSecRwRtStHdrstUpwdPosMax_Below160_Val/1 -> Mux14/2
  PA_KeSMSw4sVIPMDSecRwRtStHdrstUpwdPosMin_Below160_Val/1 -> Mux14/3
  PA_KeSMSw4sVIPMDSecRwRtStHdrstUpwdPos_Below160_Val/1 -> Mux14/1
  PA_KeSMSw4sVIPMDSecRwRtStHdrstUpwdPosMin_160_Val/1 -> Mux15/3
  PA_KeSMSw4sVIPMDSecRwRtStHdrstUpwdPosMax_160_Val/1 -> Mux15/2
  PA_KeSMSw4sVIPMDSecRwRtStHdrstUpwdPos_160_Val/1 -> Mux15/1
  PA_KeSMSw4sVIPMDSecRwRtStHdrstUpwdPosMax_165_Val/1 -> Mux16/2
  PA_KeSMSw4sVIPMDSecRwRtStHdrstUpwdPosMin_165_Val/1 -> Mux16/3
  PA_KeSMSw4sVIPMDSecRwRtStHdrstUpwdPos_165_Val/1 -> Mux16/1
  PA_KeSMSw4sVIPMDSecRwRtStHdrstUpwdPosMax_170_Val/1 -> Mux17/2
  PA_KeSMSw4sVIPMDSecRwRtStHdrstUpwdPosMin_170_Val/1 -> Mux17/3
  PA_KeSMSw4sVIPMDSecRwRtStHdrstUpwdPos_170_Val/1 -> Mux17/1
  PA_KeSMSw4sVIPMDSecRwRtStHdrstUpwdPosMax_175_Val/1 -> Mux18/2
  PA_KeSMSw4sVIPMDSecRwRtStHdrstUpwdPosMin_175_Val/1 -> Mux18/3
  PA_KeSMSw4sVIPMDSecRwRtStHdrstUpwdPos_175_Val/1 -> Mux18/1
  PA_KeSMSw4sVIPMDSecRwRtStHdrstUpwdPosMax_180_Val/1 -> Mux19/2
  PA_KeSMSw4sVIPMDSecRwRtStHdrstUpwdPosMin_180_Val/1 -> Mux19/3
  PA_KeSMSw4sVIPMDSecRwRtStHdrstUpwdPos_180_Val/1 -> Mux19/1
  PA_KeSMSw4sVIPMDSecRwRtStHdrstUpwdPosMax_Over180_Val/1 -> Mux20/2
  PA_KeSMSw4sVIPMDSecRwRtStHdrstUpwdPosMin_Over180_Val/1 -> Mux20/3
  PA_KeSMSw4sVIPMDSecRwRtStHdrstUpwdPos_Over180_Val/1 -> Mux20/1
  Mux21/1 -> Index Vector/8
  Mux22/1 -> Index Vector/7
  Mux23/1 -> Index Vector/6
  Mux24/1 -> Index Vector/5
  Mux25/1 -> Index Vector/4
  Mux26/1 -> Index Vector/3
  Mux27/1 -> Index Vector/2
  Mux/1 -> Mux27/1
  Mux1/1 -> Mux26/1
  Mux2/1 -> Mux25/1
  Mux3/1 -> Mux24/1
  Mux4/1 -> Mux23/1
  Mux5/1 -> Mux22/1
  Mux6/1 -> Mux21/1
  Mux7/1 -> Mux27/2
  Mux8/1 -> Mux26/2
  Mux9/1 -> Mux25/2
  Mux10/1 -> Mux24/2
  Mux11/1 -> Mux23/2
  Mux12/1 -> Mux22/2
  Mux13/1 -> Mux21/2
  Mux14/1 -> Mux27/3
  Mux15/1 -> Mux26/3
  Mux16/1 -> Mux25/3
  Mux17/1 -> Mux24/3
  Mux18/1 -> Mux23/3
  Mux19/1 -> Mux22/3
  Mux20/1 -> Mux21/3
  Index Vector/1 -> Demux/1
